simulink library "lib_Conduction_2DCondADI"  (R2015a)
settings: Solver=ode45  StartTime=0.0  StopTime=10.0  RelTol=1e-3
libraries: lib_GenTools_SubMatrix x24
(part 1 of 2)
settings Model: Creator=jlkratz  LastModifiedBy=jlkratz

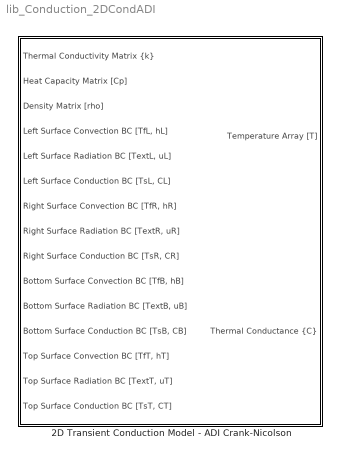
== system lib_Conduction_2DCondADI ==
  2D Transient Conduction Model - ADI Crank-Nicolson : Subsystem  mask(TSAT: 2-D Transient Conduction Model - ADI Crank-Nicolson Block){T0_M=550*ones(10,10), dt_M=1, x_M=linspace(0,3/12,10), y_M=[linspace(0,3/12,10)' linspace(0,3/12,10)' linspace(0,3/12,10)' linspace(0,3/12,10)' linspace(0,3/12,10)' linspace(0,3/12,10)' linspace(0,3/12,10)' linspace(0,3/12,10)' linspace(0,3/12,10)' linspace(0,3/12,10)'], shape_M=Planar in both directions, convL_M=on, radL_M=on, condL_M=on, convR_M=on, radR_M=on, condR_M=on, convB_M=on, radB_M=on, condB_M=on, convT_M=on, radT_M=on, condT_M=on, BN_M=double(gcb)}
      mask prompts: T0_M "T0_M - Initial temperature array [mx1]"; dt_M "dt_M - Time step [1x1]"; x_M "x_M - Discretized spatial domain in x-direction  (node locations) [nx1]"; y_M "y_M - Discretized spatial domain in r- or y-direction (node locations) [mxn]"; shape_M "shape_M - Shape in r- or y-direction"; convL_M "convL_M - Convection"; radL_M "radL_M - Radiation"; condL_M "condL_M - Conduction"; convR_M "convR_M - Convection"; radR_M "radR_M - Radiation"; condR_M "condR_M- Conduction"; convB_M "convB_M - Convection"; radB_M "radB_M - Radiation"; condB_M "condB_M - Conduction"; convT_M "convT_M - Convection"; radT_M "radT_M - Radiation"; condT_M "condT_M - Conduction"; BN_M "BN_M - Block name"
      mask help:
      | This function models the transient conduction of a 2-D structure using an alternating direction implicit (ADI) technique. It is applicable to 2-D planar and cylindrical structures. This block is able to handle variable thermal properties including density, heat capacity, and thermal conductivity. Abrupt transitions in material are also considered. It has the capability to address dynamic convection, conduction, and radiation boundary conditions. In addition, the discretized domain can be non-uniform.
      |
      | The ADI technique implemented here is NOT unconditionally stable. The chosen time-step must be suffiently small given the discretization of the structure.
      |
      | This block is able to accept inputs and parameters in a variety of units but it is important that the units be consistent. More details about this function, it's parameters, inputs, and outputs are provided in the block help menu.
      mask init:
      | %Error/Warning Checks ----------------------------------------------------%
      | 
      | % ---- x_M ---- %
      | % Not Empty?
      | if isempty(x_M) == 1
      |     fprintf('Warning in initialization of %s: x_M is an empty array.\n',char(BN_M));
      | end
      | % 1-D Array?
      | if (length(size(x_M)) ~= 2 && min(size(x_M)) ~= 1)
      |     fprintf('Warning in initialization of %s: x_M must be a 1-D array.\n',char(BN_M));
      | end
      | % Length >= 4?
      | if length(x_M) < 4
      |     fprintf('Warning in initialization of %s: x_M must have at least 4 elements.\n',char(BN_M));
      | end
      | % Real?
      | if min(isreal(x_M)) < 1
      |     fprintf('Warning in initialization of %s: x_M must have all real elements.\n',char(BN_M));
      | end
      | % Finite?
      | if min(isfinite(x_M)) < 1
      |     fprintf('Warning in initialization of %s: x_M must have all finite elements.\n',char(BN_M));
      | end
      | % All Rows Monotonically Increasing?
      | if min(diff(x_M,[],2),[],2) <= 0
      |     fprintf('Warning in initialization of %s: x_M must be monotonically increasing.\n',char(BN_M));
      | end
      | 
      | % ---- y_M ---- %
      | % Not Empty?
      | if isempty(y_M) == 1
      |     fprintf('Warning in initialization of %s: y_M is an empty array.\n',char(BN_M));
      | end
      | % 2-D Array?
      | if (length(size(y_M)) ~= 2 && min(size(y_M)) ~= 1)
      |     fprintf('Warning in initialization of %s: y_M must be a 1-D array.\n',char(BN_M));
      | end
      | % Number of rows >= 4?
      | if length(y_M) < 4
      |     fprintf('Warning in initialization of %s: y_M must have at least 4 rows.\n',char(BN_M));
      | end
      | % Real?
      | if min(isreal(y_M)) < 1
      |     fprintf('Warning in initialization of %s: y_M must have all real elements.\n',char(BN_M));
      | end
      | % Finite?
      | if min(isfinite(y_M)) < 1
      |     fprintf('Warning in initialization of %s: y_M must have all finite elements.\n',char(BN_M));
      | end
      | % All Columns are Monotonically Increasing?
      | if min(diff(y_M)) <= 0
      |     fprintf('Warning in initialization of %s: y_M must be monotonically increasing.\n',char(BN_M));
      | end
      | 
      | %Setup for simulation ----------------------------------------------------%
      | 
      | N = 20; %number of points used to integrate to find volume and 1/2 the 
      |         %points used to integrate to find J(x_M) and J(y_M)
      | 
      | %Number of rows and columns of nodes
      | m = length(y_M);
      | n = length(x_M);
      | 
      | %Natural Cubic Spline Fits
      | c = zeros(n-1,4,m);
      | for i = 1:m;
      |     c(:,:,i) = CubicSpline(x_M,y_M(i)*ones(1,n),[]);
      | end
      | 
      | %depth, dumbie value (for planar geometries only)
      | D = 1;
      | 
      | %X-DIRECTION BC PARAMETERS -----------------------------------------------%
      | 
      | %Initialize arrays
      | AL_I = zeros(1,m); %surface area of nodes on left surface
      | VL_I = zeros(1,m); %volume of nodes on the left surface
      | JLx_I = zeros(1,m); %inverse of thermal resistance * k for nodes on left surface (x-dir)
      | JLy_I = zeros(1,m-1); %inverse of thermal resistance * k for nodes on left surface (y-dir)
      | AR_I = zeros(1,m); %surface area of nodes on right surface
      | VR_I = zeros(1,m); %volume of nodes on the right surface
      | JRx_I = zeros(1,m); %inverse of thermal resistance * k for nodes on right surface (x-dir)
      | JRy_I = zeros(1,m-1); %inverse of thermal resistance * k for nodes on right surface (y-dir)
      | 
      | %LEFT SURFACE
      | j = 1;
      | for i = 1:m %for all nodes along the left surface
      |     %INTERIOR SURFACE NODE
      |     if i > 1 && i < m 
      |         %Node Corners
      |         xL = x_M(j);
      |         xR = (1/2)*(x_M(j) + x_M(j+1));
      |         yLT = (1/2)*(y_M(i) + y_M(i+1));
      |         yLB = (1/2)*(y_M(i-1) + y_M(i));
      |         yRT = (1/2)*(CubicSplineInterp( x_M,c(:,:,i+1),xR,0 ) + CubicSplineInterp( x_M,c(:,:,i),xR,0 )); 
      |         yRB = (1/2)*(CubicSplineInterp( x_M,c(:,:,i-1),xR,0 ) + CubicSplineInterp( x_M,c(:,:,i),xR,0 ));
      |         %Variable for calculating volume
      |         XV = linspace(xL,xR,N);
      |         yTXV = (1/2)*(CubicSplineInterp( x_M,c(:,:,i+1),XV,0 ) + CubicSplineInterp( x_M,c(:,:,i),XV,0 )); 
      |         yBXV = (1/2)*(CubicSplineInterp( x_M,c(:,:,i-1),XV,0 ) + CubicSplineInterp( x_M,c(:,:,i),XV,0 ));
      |         %Variables for calculating inverse of thermal resistance * k (x-dir)
      |         XJ = linspace(xL,x_M(j+1),2*N);
      |         yTXJ = (1/2)*(CubicSplineInterp( x_M,c(:,:,i+1),XJ,0 ) + CubicSplineInterp( x_M,c(:,:,i),XJ,0 ));
      |         yBXJ = (1/2)*(CubicSplineInterp( x_M,c(:,:,i-1),XJ,0 ) + CubicSplineInterp( x_M,c(:,:,i),XJ,0 ));
      |         slope = CubicSplineInterp( x_M,c(:,:,i),XJ,1 );
      |         ang = abs(atan(slope));
      |     %BOTTOM LEFT NODE
      |     elseif i == 1
      |         %Node Corners
      |         xL = x_M(j);
      |         xR = (1/2)*(x_M(j) + x_M(j+1));
      |         yLT = (1/2)*(y_M(i) + y_M(i+1));
      |         yLB = y_M(i);
      |         yRT = (1/2)*(CubicSplineInterp( x_M,c(:,:,i+1),xR,0 ) + CubicSplineInterp( x_M,c(:,:,i),xR,0 ));
      |         yRB = CubicSplineInterp( x_M,c(:,:,i),xR,0 );
      |         %Variables for calculating volume
      |         XV = linspace(xL,xR,N);
      |         yTXV = (1/2)*(CubicSplineInterp( x_M,c(:,:,i+1),XV,0 ) + CubicSplineInterp( x_M,c(:,:,i),XV,0 ));
      |         yBXV = CubicSplineInterp( x_M,c(:,:,i),XV,0 );
      |         %Variables for calculating innverse of Thermal Resistance * k
      |         XJ = linspace(xL,x_M(j+1),2*N);
      |         yTXJ = (1/2)*(CubicSplineInterp( x_M,c(:,:,i+1),XJ,0 ) + CubicSplineInterp( x_M,c(:,:,i),XJ,0 ));
      |         yBXJ = CubicSplineInterp( x_M,c(:,:,i),XJ,0 );
      |         slope = CubicSplineInterp( x_M,c(:,:,i),XJ,1 );
      |         ang = abs(atan(slope));
      |     %TOP LEFT NODE
      |     elseif i == m
      |         %Node Corners
      |         xL = x_M(j);
      |         xR = (1/2)*(x_M(j) + x_M(j+1));
      |         yLT = y_M(i);
      |         yLB = (1/2)*(y_M(i-1) + y_M(i));
      |         yRT = CubicSplineInterp( x_M,c(:,:,i),xR,0 );
      |         yRB = (1/2)*(CubicSplineInterp( x_M,c(:,:,i-1),xR,0 ) + CubicSplineInterp( x_M,c(:,:,i),xR,0 ));
      |         %Variables for calculating the volume
      |         XV = linspace(xL,xR,N);
      |         yTXV = CubicSplineInterp( x_M,c(:,:,i),XV,0 );
      |         yBXV = (1/2)*(CubicSplineInterp( x_M,c(:,:,i-1),XV,0 ) + CubicSplineInterp( x_M,c(:,:,i),XV,0 ));
      |         %Inverse of Thermal Resistance * k
      |         XJ = linspace(xL,x_M(j+1),2*N);
      |         yTXJ = CubicSplineInterp( x_M,c(:,:,i),XJ,0 );
      |         yBXJ = (1/2)*(CubicSplineInterp( x_M,c(:,:,i-1),XJ,0 ) + CubicSplineInterp( x_M,c(:,:,i),XJ,0 ));
      |         slope = CubicSplineInterp( x_M,c(:,:,i),XJ,1 );
      |         ang = abs(atan(slope));
      |     end
      |     %PLANAR IN BOTH DIRECTIONS
      |     if shape_M == 1
      |         %Area
      |         AL_I(i) = (yLT - yLB)*D;
      |         %Volume
      |         AXV = (yTXV - yBXV)*D;
      |         VL_I(i) = trapz(XV,AXV);
      |         %Inverse of Thermal Resistance * k
      |         AXJ = (yTXJ - yBXJ)*D;
      |         JLx_I(i) = trapz(XJ,1./(AXJ.*cos(ang)));
      |         if i < m
      |             AY = (xR - xL)*D;
      |             JLy_I(i) = (y_M(i+1) - y_M(i))/AY;
      |         end
      |     %PLANAR IN X-DIR, AXI-SYMMETRIC IN Y-DIR
      |     elseif shape_M == 2
      |         %Area
      |         AL_I(i) = pi*(yLT^2 - yLB^2);
      |         %Volume
      |         AXV = pi*(yTXV.^2 - yBXV.^2);
      |         VL_I(i) = trapz(XV,AXV);
      |         %Inverse of Thermal Resistance * k
      |         AXJ = pi*(yTXJ.^2 - yBXJ.^2);
      |         JLx_I(i) = trapz(XJ,1./(AXJ.*cos(ang)));
      |         if i < m
      |             Y = linspace(y_M(i),y_M(i+1),2*N);
      |             AY = 2*pi*(xR-xL)*Y;
      |             JLy_I(i) = trapz(Y,1./AY);
      |         end
      |     %AXI-SYMMETRIC IN X-DIR, PLANAR IN Y-DIR
      |     elseif shape_M == 3
      |         %Area
      |         AL_I(i) = 2*pi*xL*(yLT - yLB);
      |         %Volume
      |         AXV = 2*pi*XV'.*(yTXV - yBXV);
      |         VL_I(i) = trapz(XV,AXV);
      |         %Inverse of Thermal Resisitance * k
      |         AXJ = 2*pi*XJ'.*(yTXJ - yBXJ);
      |         JLx_I(i) = trapz(XJ,1./(AXJ.*cos(ang)));
      |         if i < m
      |             Y = linspace(y_M(i),y_M(i+1),2*N);
      |             AY = pi*(xR^2 - xL^2)*ones(1,2*N);
      |             JLy_I(i) = trapz(Y,1./AY);
      |         end
      |     end
      | end
      | 
      | %RIGHT SURFACE
      | j = n;
      | for i = 1:m %for all nodes along the right surface
      |     %INTERIOR SURFACE NODE
      |     if i > 1 && i < m 
      |         %Node Corners
      |         xL = (1/2)*(x_M(j-1) + x_M(j));
      |         xR = x_M(j);
      |         yLT = (1/2)*(CubicSplineInterp( x_M,c(:,:,i+1),xL,0 ) + CubicSplineInterp( x_M,c(:,:,i),xL,0 )); 
      |         yLB = (1/2)*(CubicSplineInterp( x_M,c(:,:,i-1),xL,0 ) + CubicSplineInterp( x_M,c(:,:,i),xL,0 ));
      |         yRT = (1/2)*(y_M(i) + y_M(i+1));
      |         yRB = (1/2)*(y_M(i-1) + y_M(i));
      |         %Variables for calculating the volume
      |         XV = linspace(xL,xR,N);
      |         yTXV = (1/2)*(CubicSplineInterp( x_M,c(:,:,i+1),XV,0 ) + CubicSplineInterp( x_M,c(:,:,i),XV,0 )); 
      |         yBXV = (1/2)*(CubicSplineInterp( x_M,c(:,:,i-1),XV,0 ) + CubicSplineInterp( x_M,c(:,:,i),XV,0 ));
      |         %Variables for calculating the inverse of Thermal Resistance * k
      |         XJ = linspace(x_M(j-1),xR,2*N);
      |         yTXJ = (1/2)*(CubicSplineInterp( x_M,c(:,:,i+1),XJ,0 ) + CubicSplineInterp( x_M,c(:,:,i),XJ,0 )); 
      |         yBXJ = (1/2)*(CubicSplineInterp( x_M,c(:,:,i-1),XJ,0 ) + CubicSplineInterp( x_M,c(:,:,i),XJ,0 ));
      |         slope = CubicSplineInterp( x_M,c(:,:,i),XJ,1 );
      |         ang = abs(atan(slope));
      |     %BOTTOM RIGHT NODE
      |     elseif i == 1
      |         %Node Corners
      |         xL = (1/2)*(x_M(j-1) + x_M(j));
      |         xR = x_M(j);
      |         yLT = (1/2)*(CubicSplineInterp( x_M,c(:,:,i+1),xL,0 ) + CubicSplineInterp( x_M,c(:,:,i),xL,0 ));
      |         yLB = CubicSplineInterp( x_M,c(:,:,i),xL,0 );
      |         yRT = (1/2)*(y_M(i) + y_M(i+1));
      |         yRB = y_M(i);
      |         %Variables for calculating the volume
      |         XV = linspace(xL,xR,N);
      |         yTXV = (1/2)*(CubicSplineInterp( x_M,c(:,:,i+1),XV,0 ) + CubicSplineInterp( x_M,c(:,:,i),XV,0 ));
      |         yBXV = CubicSplineInterp( x_M,c(:,:,i),XV,0 );
      |         %Inverse of Thermal Resistance * k
      |         XJ = linspace(x_M(j-1),xR,2*N);
      |         yTXJ = (1/2)*(CubicSplineInterp( x_M,c(:,:,i+1),XJ,0 ) + CubicSplineInterp( x_M,c(:,:,i),XJ,0 ));
      |         yBXJ = CubicSplineInterp( x_M,c(:,:,i),XJ,0 );
      |         slope = CubicSplineInterp( x_M,c(:,:,i),XJ,1 );
      |         ang = abs(atan(slope));
      |     %TOP RIGHT NODE
      |     elseif i == m
      |         %Node Corners
      |         xL = (1/2)*(x_M(j-1) + x_M(j));
      |         xR = x_M(j);
      |         yLT = CubicSplineInterp( x_M,c(:,:,i),xL,0 );
      |         yLB = (1/2)*(CubicSplineInterp( x_M,c(:,:,i-1),xL,0 ) + CubicSplineInterp( x_M,c(:,:,i),xL,0 ));
      |         yRT = y_M(i);
      |         yRB = (1/2)*(y_M(i-1) + y_M(i));
      |         %Volume
      |         XV = linspace(xL,xR,N);
      |         yTXV = CubicSplineInterp( x_M,c(:,:,i),XV,0 );
      |         yBXV = (1/2)*(CubicSplineInterp( x_M,c(:,:,i-1),XV,0 ) + CubicSplineInterp( x_M,c(:,:,i),XV,0 ));
      |         %Inverse of Thermal Resistance * k
      |         XJ = linspace(x_M(j-1),xR,2*N);
      |         yTXJ = CubicSplineInterp( x_M,c(:,:,i),XJ,0 );
      |         yBXJ = (1/2)*(CubicSplineInterp( x_M,c(:,:,i-1),XJ,0 ) + CubicSplineInterp( x_M,c(:,:,i),XJ,0 ));
      |         slope = CubicSplineInterp( x_M,c(:,:,i),XJ,1 );
      |         ang = abs(atan(slope));
      |     end
      |     %PLANAR IN BOTH DIRECTIONS
      |     if shape_M == 1
      |         %Area
      |         AR_I(i) = (yRT - yRB)*D;
      |         %Volume
      |         AXV = (yTXV - yBXV)*D;
      |         VR_I(i) = trapz(XV,AXV);
      |         %Inverse of Thermal Resistance * k
      |         AXJ = (yTXJ - yBXJ)*D;
      |         JRx_I(i) = trapz(XJ,1./(AXJ.*cos(ang)));
      |         if i < m
      |             AY = (xR - xL)*D;
      |             JRy_I(i) = (y_M(i+1) - y_M(i))/AY;
      |         end
      |     %PLANAR IN X-DIR, AXI-SYMMETRIC IN Y-DIR
      |     elseif shape_M == 2
      |         %Area
      |         AR_I(i) = pi*(yRT^2 - yRB^2);
      |         %Volume
      |         AXV = pi*(yTXV.^2 - yBXV.^2);
      |         VR_I(i) = trapz(XV,AXV);
      |         %Inverse of Thermal Resistance * k
      |         AXJ = pi*(yTXJ.^2 - yBXJ.^2);
      |         JRx_I(i) = trapz(XJ,1./(AXJ.*cos(ang)));
      |         if i < m
      |             Y = linspace(y_M(i),y_M(i+1),2*N);
      |             AY = 2*pi*(xR-xL)*Y;
      |             JRy_I(i) = trapz(Y,1./AY);
      |         end
      |     %AXI-SYMMETRIC IN X-DIR, PLANAR IN Y-DIR
      |     elseif shape_M == 3
      |         %Area
      |         AR_I(i) = 2*pi*xR*(yRT - yRB);
      |         %Volume
      |         AXV = 2*pi*XV'.*(yTXV - yBXV);
      |         VR_I(i) = trapz(XV,AXV);
      |         %Inverse of Theraml Resistance * k
      |         AXJ = 2*pi*XJ'.*(yTXJ - yBXJ);
      |         JRx_I(i) = trapz(XJ,1./(AXJ.*cos(ang)));
      |         if i < m
      |             Y = linspace(y_M(i),y_M(i+1),2*N);
      |             AY = pi*(xR^2 - xL^2)*ones(1,2*N);
      |             JRy_I(i) = trapz(Y,1./AY);
      |         end
      |     end
      | end
      | 
      | 
      | %Y-DIRECTION BC PARAMETERS -----------------------------------------------%
      | 
      | %Initialize arrays
      | AB_I = zeros(1,n); %surface area of nodes on bottom surface
      | VB_I = zeros(1,n); %volume of nodes on the bottom surface
      | JBy_I = zeros(1,n); %inverse of thermal resistance * k for nodes on bottom surface (y-dir)
      | JBx_I = zeros(1,n-1); %inverse of thermal resistance * k for nodes on bottom surface (x-dir)
      | AT_I = zeros(1,n); %surface area of nodes on top surface
      | VT_I = zeros(1,n); %volume of nodes on the top surface
      | JTy_I = zeros(1,n); %inverse of thermal resistance * k for nodes on top surface (y-dir)
      | JTx_I = zeros(1,n-1); %inverse of thermal resistance * k for nodes on top surface (x-dir)
      | 
      | %BOTTOM SURFACE
      | i = 1;
      | for j = 1:n %for all nodes along the bottom surface
      |     %INTERIOR SURFACE NODE
      |     if j > 1 && j < n
      |         %Node Corners
      |         xL = (1/2)*(x_M(j-1) + x_M(j));
      |         xR = (1/2)*(x_M(j) + x_M(j+1));
      |         yLT = (1/2)*(CubicSplineInterp( x_M,c(:,:,i+1),xL,0 ) + CubicSplineInterp( x_M,c(:,:,i),xL,0 ));
      |         yLB = CubicSplineInterp( x_M,c(:,:,i),xL,0 );
      |         yRT = (1/2)*(CubicSplineInterp( x_M,c(:,:,i+1),xR,0 ) + CubicSplineInterp( x_M,c(:,:,i),xR,0 )); 
      |         yRB = CubicSplineInterp( x_M,c(:,:,i),xR,0 );
      |         %Variable for calculating volume
      |         XV = linspace(xL,xR,N);
      |         yTXV = (1/2)*(CubicSplineInterp( x_M,c(:,:,i+1),XV,0 ) + CubicSplineInterp( x_M,c(:,:,i),XV,0 )); 
      |         yBXV = CubicSplineInterp( x_M,c(:,:,i),XV,0 );
      |     %BOTTOM LEFT NODE
      |     elseif j == 1
      |         %Node Corners
      |         xL = x_M(j);
      |         xR = (1/2)*(x_M(j) + x_M(j+1));
      |         yLT = (1/2)*(y_M(i) + y_M(i+1));
      |         yLB = y_M(i);
      |         yRT = (1/2)*(CubicSplineInterp( x_M,c(:,:,i+1),xR,0 ) + CubicSplineInterp( x_M,c(:,:,i),xR,0 ));
      |         yRB = CubicSplineInterp( x_M,c(:,:,i),xR,0 );
      |         %Variables for calculating the volume
      |         XV = linspace(xL,xR,N);
      |         yTXV = (1/2)*(CubicSplineInterp( x_M,c(:,:,i+1),XV,0 ) + CubicSplineInterp( x_M,c(:,:,i),XV,0 ));
      |         yBXV = CubicSplineInterp( x_M,c(:,:,i),XV,0 );
      |     %BOTTOM RIGHT NODE
      |     elseif j == n
      |         %Node Corners
      |         xL = (1/2)*(x_M(j-1) + x_M(j));
      |         xR = x_M(j);
      |         yLT = (1/2)*(y_M(i) + y_M(i+1));
      |         yLB = CubicSplineInterp( x_M,c(:,:,i),xL,0 );
      |         yRT = (1/2)*(CubicSplineInterp( x_M,c(:,:,i+1),xR,0 ) + CubicSplineInterp( x_M,c(:,:,i),xR,0 ));
      |         yRB = y_M(i);
      |         %Variables for calculating the volume
      |         XV = linspace(xL,xR,N);
      |         yTXV = (1/2)*(CubicSplineInterp( x_M,c(:,:,i+1),XV,0 ) + CubicSplineInterp( x_M,c(:,:,i),XV,0 ));
      |         yBXV = CubicSplineInterp( x_M,c(:,:,i),XV,0 );
      |     end
      |     %Variables for calculating the inverse of Thermal Resistance * k (in other dir)
      |     if j < n
      |         %Variables for calculating the inverse of Thermal Resistance * k
      |         XJ = linspace(x_M(j),x_M(j+1),2*N);
      |         yTXJ = (1/2)*(CubicSplineInterp( x_M,c(:,:,i+1),XJ,0 ) + CubicSplineInterp( x_M,c(:,:,i),XJ,0 )); 
      |         yBXJ = CubicSplineInterp( x_M,c(:,:,i),XJ,0 );
      |         slope = CubicSplineInterp( x_M,c(:,:,i),XJ,1 );
      |         ang = abs(atan(slope));
      |     end
      |     %PLANAR IN BOTH DIRECTIONS
      |     if shape_M == 1
      |         %Area
      |         AB_I(j) = sqrt((xR - xL)^2 + (yRB - yLB)^2)*D;
      |         %Volume
      |         AXV = (yTXV - yBXV)*D;
      |         VB_I(j) = trapz(XV,AXV);
      |         %Inverse of Thermal Resistance * k
      |         AY = (xR - xL)*D;
      |         JBy_I(j) = (y_M(i+1) - y_M(i))/AY;
      |         if j < n
      |             AXJ = (yTXJ - yBXJ)*D;
      |             JBx_I(j) = trapz(XJ,1./(AXJ.*cos(ang)));
      |         end
      |     %PLANAR IN X-DIR, AXI-SYMMETRIC IN Y-DIR
      |     elseif shape_M == 2
      |         %Area
      |         theta = abs(atan((yRB-yLB)/(xR-xL)));
      |         if theta == 0
      |             AB_I(j) = 2*pi*y_M(i)*(xR-xL);
      |         else
      |             r1 = yLB;
      |             r2 = yRB;
      |             h1 = r1/abs(tan(theta));
      |             h2 = r2/abs(tan(theta));
      |             AB_I(j) = pi*(abs(r1*sqrt(h1^2+r1^2) - r2*sqrt(h2^2+r2^2)));
      |         end
      |         %Volume
      |         AXV = pi*(yTXV.^2 - yBXV.^2);
      |         VB_I(j) = trapz(XV,AXV);
      |         %Inverse of Thermal Resistance * k
      |         Y = linspace(y_M(i),y_M(i+1),2*N);
      |         AY = 2*pi*(xR-xL)*Y;
      |         JBy_I(j) = trapz(Y,1./AY);
      |         if j < n
      |             AXJ = pi*(yTXJ.^2 - yBXJ.^2);
      |             JBx_I(j) = trapz(XJ,1./(AXJ.*cos(ang)));
      |         end
      |     %AXI-SYMMETRIC IN X-DIR, PLANAR IN Y-DIR
      |     elseif shape_M == 3
      |         %Area
      |         theta = abs(atan((yRB-yLB)/(xR-xL)));
      |         if theta == 0
      |             AB_I(j) = pi*(xR^2-xL^2);
      |         else
      |             r1 = xR;
      |             r2 = xL;
      |             h1 = r1*abs(tan(theta));
      |             h2 = r2*abs(tan(theta));
      |             AB_I(j) = pi*(abs(r1*sqrt(h1^2+r1^2) - r2*sqrt(h2^2+r2^2)));
      |         end
      |         %Volume
      |         AXV = 2*pi*XV'.*(yTXV - yBXV);
      |         VB_I(j) = trapz(XV,AXV); 
      |         %Inverse of Thermal Resistance * k
      |         Y = linspace(y_M(i),y_M(i+1),2*N);
      |         AY = pi*(xR^2 - xL^2)*ones(1,2*N);
      |         JBy_I(j) = trapz(Y,1./AY);
      |         if j < n
      |             AXJ = 2*pi*XJ'.*(yTXJ - yBXJ);
      |             JBx_I(j) = trapz(XJ,1./(AXJ.*cos(ang)));
      |         end
      |     end
      | end
      | 
      | %TOP SURFACE
      | i = m;
      | for j = 1:n %for all nodes along the top surface
      |     %INTERIOR SURFACE NODE
      |     if j > 1 && j < n
      |         %Node Corners
      |         xL = (1/2)*(x_M(j-1) + x_M(j));
      |         xR = (1/2)*(x_M(j) + x_M(j+1));
      |         yLT = CubicSplineInterp( x_M,c(:,:,i),xL,0 );
      |         yLB = (1/2)*(CubicSplineInterp( x_M,c(:,:,i-1),xL,0 ) + CubicSplineInterp( x_M,c(:,:,i),xL,0 ));
      |         yRT = CubicSplineInterp( x_M,c(:,:,i),xR,0 );
      |         yRB = (1/2)*(CubicSplineInterp( x_M,c(:,:,i-1),xR,0 ) + CubicSplineInterp( x_M,c(:,:,i),xR,0 ));
      |         %Variables for calculating the volume
      |         XV = linspace(xL,xR,N);
      |         yTXV = CubicSplineInterp( x_M,c(:,:,i),XV,0 );
      |         yBXV = (1/2)*(CubicSplineInterp( x_M,c(:,:,i-1),XV,0 ) + CubicSplineInterp( x_M,c(:,:,i),XV,0 ));
      |     %TOP LEFT NODE
      |     elseif j == 1
      |         %Node Corners
      |         xL = x_M(j);
      |         xR = (1/2)*(x_M(j) + x_M(j+1));
      |         yLT = y_M(i);
      |         yLB = (1/2)*(y_M(i) + y_M(i-1));
      |         yRT = CubicSplineInterp( x_M,c(:,:,i),xR,0 );
      |         yRB = (1/2)*(CubicSplineInterp( x_M,c(:,:,i-1),xR,0 ) + CubicSplineInterp( x_M,c(:,:,i),xR,0 ));
      |         %Variables for calculating the volume
      |         XV = linspace(xL,xR,N);
      |         yTXV = CubicSplineInterp( x_M,c(:,:,i),XV,0 );
      |         yBXV = (1/2)*(CubicSplineInterp( x_M,c(:,:,i-1),XV,0 ) + CubicSplineInterp( x_M,c(:,:,i),XV,0 ));
      |     %TOP RIGHT NODE
      |     elseif j == n
      |         %Node Corners
      |         xL = (1/2)*(x_M(j-1) + x_M(j));
      |         xR = x_M(j);
      |         yLT = CubicSplineInterp( x_M,c(:,:,i),xL,0 );
      |         yLB = (1/2)*(CubicSplineInterp( x_M,c(:,:,i-1),xL,0 ) + CubicSplineInterp( x_M,c(:,:,i),xL,0 ));
      |         yRT = y_M(i);
      |         yRB = (1/2)*(y_M(i-1) + y_M(i));
      |         %Volume
      |         XV = linspace(xL,xR,N);
      |         yTXV = CubicSplineInterp( x_M,c(:,:,i),XV,0 );
      |         yBXV = (1/2)*(CubicSplineInterp( x_M,c(:,:,i-1),XV,0 ) + CubicSplineInterp( x_M,c(:,:,i),XV,0 ));
      |     end
      |     %Variables for calculating the inverse of Thermal Resistance * k (in other dir)
      |     if j < n
      |         %Variables for calculating the inverse of Thermal Resistance * k
      |         XJ = linspace(x_M(j),x_M(j+1),2*N);
      |         yTXJ = CubicSplineInterp( x_M,c(:,:,i),XJ,0 ); 
      |         yBXJ = (1/2)*(CubicSplineInterp( x_M,c(:,:,i-1),XJ,0 ) + CubicSplineInterp( x_M,c(:,:,i),XJ,0 ));
      |         slope = CubicSplineInterp( x_M,c(:,:,i),XJ,1 );
      |         ang = abs(atan(slope));
      |     end
      |     %PLANAR IN BOTH DIRECTIONS
      |     if shape_M == 1
      |         %Area
      |         AT_I(j) = sqrt((xR - xL)^2 + (yRT - yLT)^2)*D;
      |         %Volume
      |         AXV = (yTXV - yBXV)*D;
      |         VT_I(j) = trapz(XV,AXV);
      |         %Inverse of Thermal Resistance * k
      |         AY = (xR - xL)*D;
      |         JTy_I(j) = (y_M(i) - y_M(i-1))/AY;
      |         if j < n
      |             AXJ = (yTXJ - yBXJ)*D;
      |             JTx_I(j) = trapz(XJ,1./(AXJ.*cos(ang)));
      |         end
      |     %PLANAR IN X-DIR, AXI-SYMMETRIC IN Y-DIR
      |     elseif shape_M == 2
      |         %Area
      |         theta = abs(atan((yRT-yLT)/(xR-xL)));
      |         if theta == 0
      |             AT_I(j) = 2*pi*y_M(i)*(xR-xL);
      |         else
      |             r1 = yLT;
      |             r2 = yRT;
      |             h1 = r1/abs(tan(theta));
      |             h2 = r2/abs(tan(theta));
      |             AT_I(j) = pi*(abs(r1*sqrt(h1^2+r1^2) - r2*sqrt(h2^2+r2^2)));
      |         end
      |         %Volume
      |         AXV = pi*(yTXV.^2 - yBXV.^2);
      |         VT_I(j) = trapz(XV,AXV);
      |         %Inverse of Thermal Resistance * k
      |         Y = linspace(y_M(i-1),y_M(i),2*N);
      |         AY = 2*pi*(xR-xL)*Y;
      |         JTy_I(j) = trapz(Y,1./AY);
      |         if j < n
      |             AXJ = pi*(yTXJ.^2 - yBXJ.^2);
      |             JTx_I(j) = trapz(XJ,1./(AXJ.*cos(ang)));
      |         end
      |     %AXI-SYMMETRIC IN X-DIR, PLANAR IN Y-DIR
      |     elseif shape_M == 3
      |         %Area
      |         theta = abs(atan((yRT-yLT)/(xR-xL)));
      |         if theta == 0
      |             AT_I(j) = pi*(xR^2-xL^2);
      |         else
      |             r1 = xR;
      |             r2 = xL;
      |             h1 = r1*abs(tan(theta));
      |             h2 = r2*abs(tan(theta));
      |             AT_I(j) = pi*(abs(r1*sqrt(h1^2+r1^2) - r2*sqrt(h2^2+r2^2)));
      |         end
      |         %Volume
      |         AXV = 2*pi*XV'.*(yTXV - yBXV);
      |         VT_I(j) = trapz(XV,AXV); 
      |         %Inverse of Thermal Resistance * k
      |         Y = linspace(y_M(i-1),y_M(i),2*N);
      |         AY = pi*(xR^2 - xL^2)*ones(1,2*N);
      |         JTy_I(j) = trapz(Y,1./AY);
      |         if j < n
      |             AXJ = 2*pi*XJ'.*(yTXJ - yBXJ);
      |             JTx_I(j) = trapz(XJ,1./(AXJ.*cos(ang)));
      |         end
      |     end
      | end
      | 
      | % Setup Inports ----------------------------------------------------------%
      | 
      | % Inport Numbers
      | n = 4; %first BC inport number
      | 
      | % Left Surface Convection Boundary Condition
      | if convL_M == 1
      |     if strcmp(get_param([BN_M '/Left Surface Convection BC [TfL, hL]'],'BlockType'),'Constant')
      |         MSK_ReplaceBlock_TSAT([BN_M '/Left Surface Convection BC [TfL, hL]'],'built-in/Inport');
      |     end
      |     set_param([BN_M '/Left Surface Convection BC [TfL, hL]'],'Port',num2str(n));
      |     n = n + 1;
      | elseif convL_M == 0
      |     if strcmp(get_param([BN_M '/Left Surface Convection BC [TfL, hL]'],'BlockType'),'Inport')
      |         MSK_ReplaceBlock_TSAT([BN_M '/Left Surface Convection BC [TfL, hL]'],'built-in/Constant');
      |         set_param([BN_M '/Left Surface Convection BC [TfL, hL]'],'Value','zeros(length(y_M),2)');
      |     end
      | end
      | 
      | % Left Surface Radiation Boundary Condition
      | if radL_M == 1
      |     if strcmp(get_param([BN_M '/Left Surface Radiation BC [TextL, uL]'],'BlockType'),'Constant')
      |         MSK_ReplaceBlock_TSAT([BN_M '/Left Surface Radiation BC [TextL, uL]'],'built-in/Inport');
      |     end
      |     set_param([BN_M '/Left Surface Radiation BC [TextL, uL]'],'Port',num2str(n));
      |     n = n + 1;
      | elseif radL_M == 0
      |     if strcmp(get_param([BN_M '/Left Surface Radiation BC [TextL, uL]'],'BlockType'),'Inport')
      |         MSK_ReplaceBlock_TSAT([BN_M '/Left Surface Radiation BC [TextL, uL]'],'built-in/Constant');
      |         set_param([BN_M '/Left Surface Radiation BC [TextL, uL]'],'Value','zeros(length(y_M),2)');
      |     end
      | end
      | 
      | % Left Surface Conduction Boundary Condition
      | if condL_M == 1
      |     if strcmp(get_param([BN_M '/Left Surface Conduction BC [TsL, CL]'],'BlockType'),'Constant')
      |         MSK_ReplaceBlock_TSAT([BN_M '/Left Surface Conduction BC [TsL, CL]'],'built-in/Inport');
      |     end
      |     set_param([BN_M '/Left Surface Conduction BC [TsL, CL]'],'Port',num2str(n));
      |     n = n + 1;
      | elseif condL_M == 0
      |     if strcmp(get_param([BN_M '/Left Surface Conduction BC [TsL, CL]'],'BlockType'),'Inport')
      |         MSK_ReplaceBlock_TSAT([BN_M '/Left Surface Conduction BC [TsL, CL]'],'built-in/Constant');
      |         set_param([BN_M '/Left Surface Conduction BC [TsL, CL]'],'Value','zeros(length(y_M),2)');
      |     end
      | end
      | 
      | % Right Surface Convection Boundary Condition
      | if convR_M == 1
      |     if strcmp(get_param([BN_M '/Right Surface Convection BC [TfR, hR]'],'BlockType'),'Constant')
      |         MSK_ReplaceBlock_TSAT([BN_M '/Right Surface Convection BC [TfR, hR]'],'built-in/Inport');
      |     end
      |     set_param([BN_M '/Right Surface Convection BC [TfR, hR]'],'Port',num2str(n));
      |     n = n + 1;
      | elseif convR_M == 0
      |     if strcmp(get_param([BN_M '/Right Surface Convection BC [TfR, hR]'],'BlockType'),'Inport')
      |         MSK_ReplaceBlock_TSAT([BN_M '/Right Surface Convection BC [TfR, hR]'],'built-in/Constant');
      |         set_param([BN_M '/Right Surface Convection BC [TfR, hR]'],'Value','zeros(length(y_M),2)');
      |     end
      | end
      | 
      | % Right Surface Radiation Boundary Condition
      | if radR_M == 1
      |     if strcmp(get_param([BN_M '/Right Surface Radiation BC [TextR, uR]'],'BlockType'),'Constant')
      |         MSK_ReplaceBlock_TSAT([BN_M '/Right Surface Radiation BC [TextR, uR]'],'built-in/Inport');
      |     end
      |     set_param([BN_M '/Right Surface Radiation BC [TextR, uR]'],'Port',num2str(n));
      |     n = n + 1;
      | elseif radR_M == 0
      |     if strcmp(get_param([BN_M '/Right Surface Radiation BC [TextR, uR]'],'BlockType'),'Inport')
      |         MSK_ReplaceBlock_TSAT([BN_M '/Right Surface Radiation BC [TextR, uR]'],'built-in/Constant');
      |         set_param([BN_M '/Right Surface Radiation BC [TextR, uR]'],'Value','zeros(length(y_M),2)');
      |     end
      | end
      | 
      | % Right Surface Conduction Boundary Condition
      | if condR_M == 1
      |     if strcmp(get_param([BN_M '/Right Surface Conduction BC [TsR, CR]'],'BlockType'),'Constant')
      |         MSK_ReplaceBlock_TSAT([BN_M '/Right Surface Conduction BC [TsR, CR]'],'built-in/Inport');
      |     end
      |     set_param([BN_M '/Right Surface Conduction BC [TsR, CR]'],'Port',num2str(n));
      |     n = n + 1;
      | elseif condR_M == 0
      |     if strcmp(get_param([BN_M '/Right Surface Conduction BC [TsR, CR]'],'BlockType'),'Inport')
      |         MSK_ReplaceBlock_TSAT([BN_M '/Right Surface Conduction BC [TsR, CR]'],'built-in/Constant');
      |         set_param([BN_M '/Right Surface Conduction BC [TsR, CR]'],'Value','zeros(length(y_M),2)');
      |     end
      | end
      | 
      | % Bottom Surface Convection Boundary Condition
      | if convB_M == 1
      |     if strcmp(get_param([BN_M '/Bottom Surface Convection BC [TfB, hB]'],'BlockType'),'Constant')
      |         MSK_ReplaceBlock_TSAT([BN_M '/Bottom Surface Convection BC [TfB, hB]'],'built-in/Inport');
      |     end
      |     set_param([BN_M '/Bottom Surface Convection BC [TfB, hB]'],'Port',num2str(n));
      |     n = n + 1;
      | elseif convB_M == 0
      |     if strcmp(get_param([BN_M '/Bottom Surface Convection BC [TfB, hB]'],'BlockType'),'Inport')
      |         MSK_ReplaceBlock_TSAT([BN_M '/Bottom Surface Convection BC [TfB, hB]'],'built-in/Constant');
      |         set_param([BN_M '/Bottom Surface Convection BC [TfB, hB]'],'Value','zeros(length(x_M),2)');
      |     end
      | end
      | 
      | % Bottom Surface Radiation Boundary Condition
      | if radB_M == 1
      |     if strcmp(get_param([BN_M '/Bottom Surface Radiation BC [TextB, uB]'],'BlockType'),'Constant')
      |         MSK_ReplaceBlock_TSAT([BN_M '/Bottom Surface Radiation BC [TextB, uB]'],'built-in/Inport');
      |     end
      |     set_param([BN_M '/Bottom Surface Radiation BC [TextB, uB]'],'Port',num2str(n));
      |     n = n + 1;
      | elseif radB_M == 0
      |     if strcmp(get_param([BN_M '/Bottom Surface Radiation BC [TextB, uB]'],'BlockType'),'Inport')
      |         MSK_ReplaceBlock_TSAT([BN_M '/Bottom Surface Radiation BC [TextB, uB]'],'built-in/Constant');
      |         set_param([BN_M '/Bottom Surface Radiation BC [TextB, uB]'],'Value','zeros(length(x_M),2)');
      |     end
      | end
      | 
      | % Bottom Surface Conduction Boundary Condition
      | if condB_M == 1
      |     if strcmp(get_param([BN_M '/Bottom Surface Conduction BC [TsB, CB]'],'BlockType'),'Constant')
      |         MSK_ReplaceBlock_TSAT([BN_M '/Bottom Surface Conduction BC [TsB, CB]'],'built-in/Inport');
      |     end
      |     set_param([BN_M '/Bottom Surface Conduction BC [TsB, CB]'],'Port',num2str(n));
      |     n = n + 1;
      | elseif condB_M == 0
      |     if strcmp(get_param([BN_M '/Bottom Surface Conduction BC [TsB, CB]'],'BlockType'),'Inport')
      |         MSK_ReplaceBlock_TSAT([BN_M '/Bottom Surface Conduction BC [TsB, CB]'],'built-in/Constant');
      |         set_param([BN_M '/Bottom Surface Conduction BC [TsB, CB]'],'Value','zeros(length(x_M),2)');
      |     end
      | end
      | 
      | % Top Surface Convection Boundary Condition
      | if convT_M == 1
      |     if strcmp(get_param([BN_M '/Top Surface Convection BC [TfT, hT]'],'BlockType'),'Constant')
      |         MSK_ReplaceBlock_TSAT([BN_M '/Top Surface Convection BC [TfT, hT]'],'built-in/Inport');
      |     end
      |     set_param([BN_M '/Top Surface Convection BC [TfT, hT]'],'Port',num2str(n));
      |     n = n + 1;
      | elseif convT_M == 0
      |     if strcmp(get_param([BN_M '/Top Surface Convection BC [TfT, hT]'],'BlockType'),'Inport')
      |         MSK_ReplaceBlock_TSAT([BN_M '/Top Surface Convection BC [TfT, hT]'],'built-in/Constant');
      |         set_param([BN_M '/Top Surface Convection BC [TfT, hT]'],'Value','zeros(length(x_M),2)');
      |     end
      | end
      | 
      | % Top Surface Radiation Boundary Condition
      | if radT_M == 1
      |     if strcmp(get_param([BN_M '/Top Surface Radiation BC [TextT, uT]'],'BlockType'),'Constant')
      |         MSK_ReplaceBlock_TSAT([BN_M '/Top Surface Radiation BC [TextT, uT]'],'built-in/Inport');
      |     end
      |     set_param([BN_M '/Top Surface Radiation BC [TextT, uT]'],'Port',num2str(n));
      |     n = n + 1;
      | elseif radT_M == 0
      |     if strcmp(get_param([BN_M '/Top Surface Radiation BC [TextT, uT]'],'BlockType'),'Inport')
      |         MSK_ReplaceBlock_TSAT([BN_M '/Top Surface Radiation BC [TextT, uT]'],'built-in/Constant');
      |         set_param([BN_M '/Top Surface Radiation BC [TextT, uT]'],'Value','zeros(length(x_M),2)');
      |     end
      | end
      | 
      | % Top Surface Conduction Boundary Condition
      | if condT_M == 1
      |     if strcmp(get_param([BN_M '/Top Surface Conduction BC [TsT, CT]'],'BlockType'),'Constant')
      |         MSK_ReplaceBlock_TSAT([BN_M '/Top Surface Conduction BC [TsT, CT]'],'built-in/Inport');
      |     end
      |     set_param([BN_M '/Top Surface Conduction BC [TsT, CT]'],'Port',num2str(n));
      |     n = n + 1;
      | elseif condT_M == 0
      |     if strcmp(get_param([BN_M '/Top Surface Conduction BC [TsT, CT]'],'BlockType'),'Inport')
      |         MSK_ReplaceBlock_TSAT([BN_M '/Top Surface Conduction BC [TsT, CT]'],'built-in/Constant');
      |         set_param([BN_M '/Top Surface Conduction BC [TsT, CT]'],'Value','zeros(length(x_M),2)');
      |     end
      | end
      mask Help: web(which('Conduction_TSAT_2DCondADI.html'),'-helpbrowser')
      mask TypeOptions shape_M: Planar in both directions | Planar in x-direction, Axi-symmetric in y-direction | Axi-Symmetric in x-direction, Planar in y-direction
      mask DialogControl Container3 Prompt: General Parameters
      mask DialogControl Container6 Prompt: Geometry
      mask DialogControl Container4 Prompt: Active Left Boundary Conditions
      mask DialogControl Container7 Prompt: Active Right Boundary Conditions
      mask DialogControl Container9 Prompt: Active Bottom Boundary Condidions
      mask DialogControl Container11 Prompt: Active Top Boundary Conditions

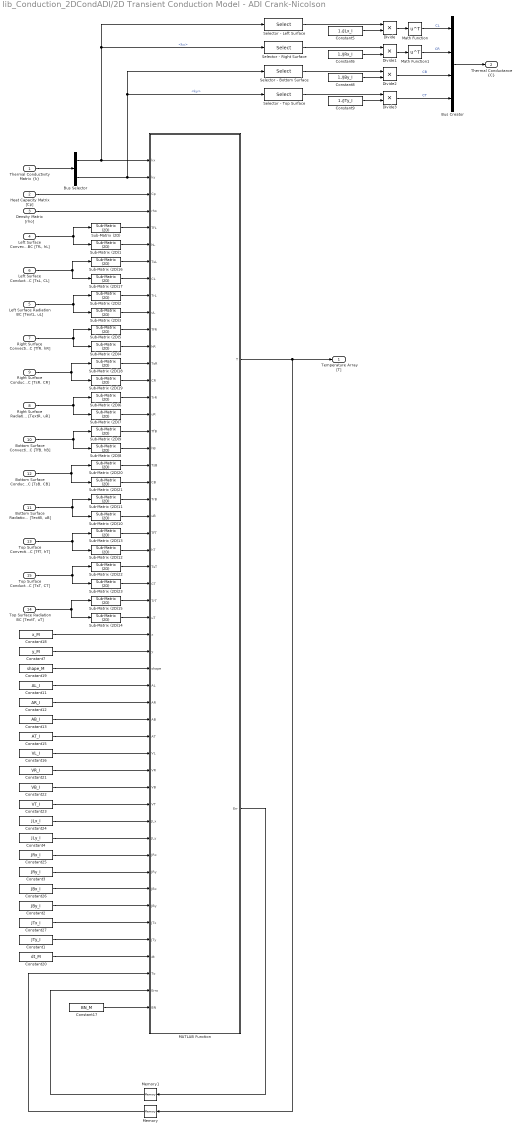
== system lib_Conduction_2DCondADI/2D Transient Conduction Model - ADI Crank-Nicolson ==
  "Thermal Conductivity Matrix {k}" : Inport
  Heat Capacity Matrix [Cp] : Inport  Port=2
  Density Matrix [rho] : Inport  Port=3
  "Left Surface Convection BC [TfL, hL]" : Inport  Port=4
  "Left Surface Radiation BC [TextL, uL]" : Inport  Port=5
  "Left Surface Conduction BC [TsL, CL]" : Inport  Port=6
  "Right Surface Convection BC [TfR, hR]" : Inport  Port=7
  "Right Surface Radiation BC [TextR, uR]" : Inport  Port=8
  "Right Surface Conduction BC [TsR, CR]" : Inport  Port=9
  "Bottom Surface Convection BC [TfB, hB]" : Inport  Port=10
  "Bottom Surface Radiation BC [TextB, uB]" : Inport  Port=11
  "Bottom Surface Conduction BC [TsB, CB]" : Inport  Port=12
  "Top Surface Convection BC [TfT, hT]" : Inport  Port=13
  "Top Surface Radiation BC [TextT, uT]" : Inport  Port=14
  "Top Surface Conduction BC [TsT, CT]" : Inport  Port=15
  Bus Creator : BusCreator
  Bus Selector : BusSelector  OutputSignals=kx,ky
  Constant1 : Constant  Value=JTy_I
  Constant11 : Constant  Value=AL_I
  Constant12 : Constant  Value=AR_I
  Constant13 : Constant  Value=AB_I
  Constant15 : Constant  Value=AT_I
  Constant16 : Constant  Value=VL_I
  Constant17 : Constant  Value=BN_M
  Constant18 : Constant  Value=x_M
  Constant19 : Constant  Value=shape_M
  Constant2 : Constant  Value=JBy_I
  Constant20 : Constant  Value=dt_M
  Constant21 : Constant  Value=VR_I
  Constant22 : Constant  Value=VB_I
  Constant23 : Constant  Value=VT_I
  Constant24 : Constant  Value=JLx_I
  Constant25 : Constant  Value=JRx_I
  Constant26 : Constant  Value=JBx_I
  Constant27 : Constant  Value=JTx_I
  Constant3 : Constant  Value=JRy_I
  Constant4 : Constant  Value=JLy_I
  Constant5 : Constant  Value=1./JLx_I
  Constant6 : Constant  Value=1./JRx_I
  Constant7 : Constant  Value=y_M
  Constant8 : Constant  Value=1./JBy_I
  Constant9 : Constant  Value=1./JTy_I
  Divide{,1..3} (4 alike) : Product  Inputs=**
  MATLAB Function : MATLAB Function  TreatAsAtomicUnit=on
  Math Function : Math  Operator=transpose  SaturateOnIntegerOverflow=on
  Math Function1 : Math  Operator=transpose  SaturateOnIntegerOverflow=on
  Memory : Memory  X0=T0_M
  Memory1 : Memory  X0=zeros(1,180)
  Selector - Bottom Surface : Selector  NumberOfDimensions=2  InputPortWidth=3  IndexOptions=Index vector (dialog),Select all  Indices=1,1  OutputSizes=1,1
  Selector - Left Surface : Selector  NumberOfDimensions=2  InputPortWidth=3  IndexOptions=Select all,Index vector (dialog)  Indices=,1  OutputSizes=1,1
  Selector - Right Surface : Selector  NumberOfDimensions=2  InputPortWidth=3  IndexOptions=Select all,Index vector (dialog)  Indices=,length(x_M)  OutputSizes=1,1
  Selector - Top Surface : Selector  NumberOfDimensions=2  InputPortWidth=3  IndexOptions=Index vector (dialog),Select all  Indices=length(y_M),1  OutputSizes=1,1
  Sub-Matrix (2D){,2,5..6,16,18} (6 alike) : lib_GenTools_SubMatrix/Sub-Matrix (2D)  R1_M=1  R2_M=length(y_M)  C1_M=1  C2_M=1  BN_M=double(gcb)
  Sub-Matrix (2D){1,3..4,7,17,19} (6 alike) : lib_GenTools_SubMatrix/Sub-Matrix (2D)  R1_M=1  R2_M=length(y_M)  C1_M=2  C2_M=2  BN_M=double(gcb)
  Sub-Matrix (2D){8,10,12,14,21,23} (6 alike) : lib_GenTools_SubMatrix/Sub-Matrix (2D)  R1_M=1  R2_M=length(x_M)  C1_M=2  C2_M=2  BN_M=double(gcb)
  Sub-Matrix (2D){9,11,13,15,20,22} (6 alike) : lib_GenTools_SubMatrix/Sub-Matrix (2D)  R1_M=1  R2_M=length(x_M)  C1_M=1  C2_M=1  BN_M=double(gcb)
  Temperature Array [T] : Outport
  "Thermal Conductance {C}" : Outport  Port=2
  wires:
  Constant13/1 -> MATLAB Function/34(AB)
  Constant1/1 -> MATLAB Function/47(JTy)
  Constant27/1 -> MATLAB Function/46(JTx)
  Constant2/1 -> MATLAB Function/45(JBy)
  Constant26/1 -> MATLAB Function/44(JBx)
  Constant3/1 -> MATLAB Function/43(JRy)
  Constant25/1 -> MATLAB Function/42(JRx)
  Constant4/1 -> MATLAB Function/41(JLy)
  "Right Surface Radiation BC [TextR, uR]"/1 -> Sub-Matrix (2D)7/1, Sub-Matrix (2D)6/1
  Sub-Matrix (2D)7/1 -> MATLAB Function/16(uR)
  Sub-Matrix (2D)6/1 -> MATLAB Function/15(TrR)
  Sub-Matrix (2D)4/1 -> MATLAB Function/12(hR)
  Sub-Matrix (2D)3/1 -> MATLAB Function/10(uL)
  Sub-Matrix (2D)2/1 -> MATLAB Function/9(TrL)
  "Left Surface Radiation BC [TextL, uL]"/1 -> Sub-Matrix (2D)3/1, Sub-Matrix (2D)2/1
  Sub-Matrix (2D)1/1 -> MATLAB Function/6(hL)
  Sub-Matrix (2D)/1 -> MATLAB Function/5(TfL)
  "Left Surface Convection BC [TfL, hL]"/1 -> Sub-Matrix (2D)1/1, Sub-Matrix (2D)/1
  MATLAB Function/2(Err) -> Memory1/1
  Memory/1 -> MATLAB Function/49(To)
  MATLAB Function/1(T) -> Memory/1, Temperature Array [T]/1
  Constant20/1 -> MATLAB Function/48(dt)
  Constant19/1 -> MATLAB Function/31(shape)
  Constant18/1 -> MATLAB Function/29(x)
  Density Matrix [rho]/1 -> MATLAB Function/4(rho)
  Heat Capacity Matrix [Cp]/1 -> MATLAB Function/3(Cp)
  Memory1/1 -> MATLAB Function/50(Erro)
  Constant17/1 -> MATLAB Function/51(BN)
  "Top Surface Radiation BC [TextT, uT]"/1 -> Sub-Matrix (2D)14/1, Sub-Matrix (2D)15/1
  Sub-Matrix (2D)14/1 -> MATLAB Function/28(uT)
  Sub-Matrix (2D)15/1 -> MATLAB Function/27(TrT)
  Sub-Matrix (2D)12/1 -> MATLAB Function/24(hT)
  Sub-Matrix (2D)13/1 -> MATLAB Function/23(TfT)
  "Top Surface Convection BC [TfT, hT]"/1 -> Sub-Matrix (2D)13/1, Sub-Matrix (2D)12/1
  Sub-Matrix (2D)10/1 -> MATLAB Function/22(uB)
  Sub-Matrix (2D)11/1 -> MATLAB Function/21(TrB)
  "Bottom Surface Radiation BC [TextB, uB]"/1 -> Sub-Matrix (2D)10/1, Sub-Matrix (2D)11/1
  Sub-Matrix (2D)8/1 -> MATLAB Function/18(hB)
  Sub-Matrix (2D)9/1 -> MATLAB Function/17(TfB)
  "Bottom Surface Convection BC [TfB, hB]"/1 -> Sub-Matrix (2D)8/1, Sub-Matrix (2D)9/1
  Constant7/1 -> MATLAB Function/30(y)
  Sub-Matrix (2D)5/1 -> MATLAB Function/11(TfR)
  "Right Surface Convection BC [TfR, hR]"/1 -> Sub-Matrix (2D)5/1, Sub-Matrix (2D)4/1
  Divide/1 -> Math Function/1
  Divide1/1 -> Math Function1/1
  Divide2/1 -> Bus Creator/3  "CB"
  Divide3/1 -> Bus Creator/4  "CT"
  Bus Creator/1 -> "Thermal Conductance {C}"/1
  Selector - Right Surface/1 -> Divide1/1
  Constant5/1 -> Divide/2
  Selector - Left Surface/1 -> Divide/1
  Constant6/1 -> Divide1/2
  Selector - Bottom Surface/1 -> Divide2/1
  Selector - Top Surface/1 -> Divide3/1
  Constant8/1 -> Divide2/2
  Constant9/1 -> Divide3/2
  Constant11/1 -> MATLAB Function/32(AL)
  Constant12/1 -> MATLAB Function/33(AR)
  Constant15/1 -> MATLAB Function/35(AT)
  Constant21/1 -> MATLAB Function/37(VR)
  Constant22/1 -> MATLAB Function/38(VB)
  Constant24/1 -> MATLAB Function/40(JLx)
  Bus Selector/2 -> Selector - Top Surface/1, Selector - Bottom Surface/1, MATLAB Function/2(ky)  "<ky>"
  Bus Selector/1 -> Selector - Right Surface/1, Selector - Left Surface/1, MATLAB Function/1(kx)  "<kx>"
  "Thermal Conductivity Matrix {k}"/1 -> Bus Selector/1
  "Left Surface Conduction BC [TsL, CL]"/1 -> Sub-Matrix (2D)17/1, Sub-Matrix (2D)16/1
  "Right Surface Conduction BC [TsR, CR]"/1 -> Sub-Matrix (2D)18/1, Sub-Matrix (2D)19/1
  "Bottom Surface Conduction BC [TsB, CB]"/1 -> Sub-Matrix (2D)20/1, Sub-Matrix (2D)21/1
  "Top Surface Conduction BC [TsT, CT]"/1 -> Sub-Matrix (2D)23/1, Sub-Matrix (2D)22/1
  Sub-Matrix (2D)23/1 -> MATLAB Function/26(CT)
  Sub-Matrix (2D)22/1 -> MATLAB Function/25(TsT)
  Sub-Matrix (2D)21/1 -> MATLAB Function/20(CB)
  Sub-Matrix (2D)20/1 -> MATLAB Function/19(TsB)
  Sub-Matrix (2D)19/1 -> MATLAB Function/14(CR)
  Sub-Matrix (2D)18/1 -> MATLAB Function/13(TsR)
  Sub-Matrix (2D)17/1 -> MATLAB Function/8(CL)
  Sub-Matrix (2D)16/1 -> MATLAB Function/7(TsL)
  Math Function/1 -> Bus Creator/1  "CL"
  Math Function1/1 -> Bus Creator/2  "CR"
  Constant16/1 -> MATLAB Function/36(VL)
  Constant23/1 -> MATLAB Function/39(VT)
